simulink model "crazyflie"  (R2015b)
settings: Solver=FixedStepAuto  StartTime=0.0  StopTime=18  FixedStep=1/500  MinStep=1e-4  RelTol=1e-3
undefined symbols (not defined in the file): A, B, C, D
libraries: simulink x1
(part 1 of 3)
settings Model: NumberOfSteps=250  Creator=mattcollins  LastModifiedBy=mattcollins
settings SolverCC: AutoInsertRateTranBlk=on

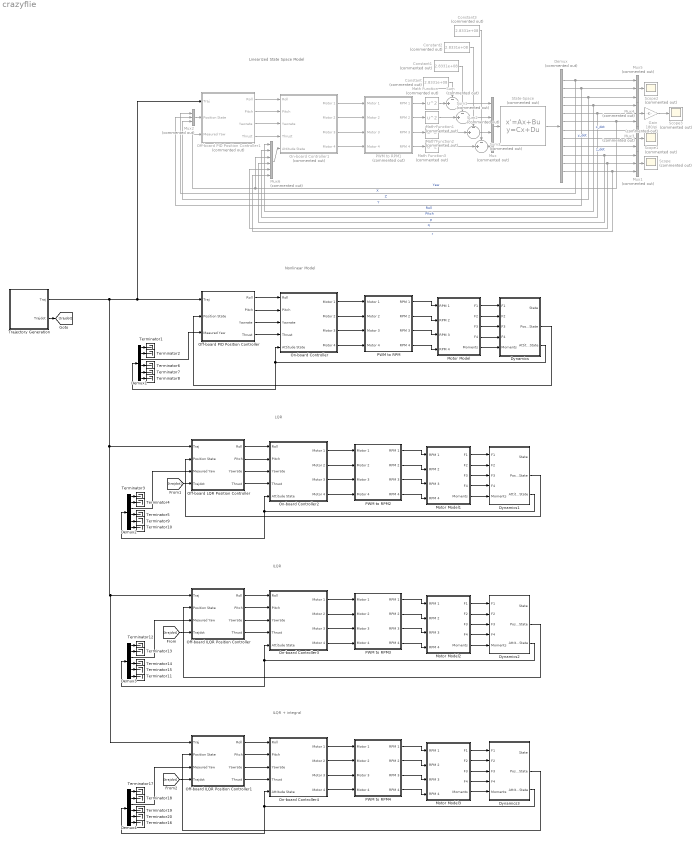
== system crazyflie ==
  note: Nonlinear Model
  note: Linearized State Space Model
  note: LQR
  note: ILQR
  note: ILQR + integral
  Constant{,1..3} (4 alike) : Constant  Commented=on  Value=2.8331e+08
  Demux : Demux  Commented=on  Outputs=12
  Demux{1..4} (4 alike) : Demux  Outputs=6
  Dynamics : Subsystem
  Dynamics1 : Subsystem
  Dynamics2 : Subsystem
  Dynamics3 : Subsystem
  Gain : Gain  Commented=on  Gain=180/pi
  Math Function{,1..3} (4 alike) : Math  Commented=on  Operator=square  SaturateOnIntegerOverflow=on
  Motor Model : Subsystem
  Motor Model1 : Subsystem
  Motor Model2 : Subsystem
  Motor Model3 : Subsystem
  Mux : Mux  Commented=on
  Mux{1..5} (5 alike) : Mux  Commented=on  Inputs=3
  Mux6 : Mux  Commented=on  Inputs=6
  Off-board ILQR Position Controller : Subsystem
  Off-board ILQR Position Controller1 : Subsystem
  "Off-board LQR Position Controller " : Subsystem
  Off-board PID Position Controller : Subsystem
  Off-board PID Position Controller1 : Subsystem  Commented=on
  On-board Controller : Subsystem
  On-board Controller1 : Subsystem  Commented=on
  On-board Controller2 : Subsystem
  On-board Controller3 : Subsystem
  On-board Controller4 : Subsystem
  PWM to RPM : Subsystem
  PWM to RPM1 : Subsystem  Commented=on
  PWM to RPM2 : Subsystem
  PWM to RPM3 : Subsystem
  PWM to RPM4 : Subsystem
  Scope{,1..3} (4 alike) : Scope  Commented=on
  State-Space : StateSpace  Commented=on  A=A  B=B  C=C  D=D  X0=[0;0;1;0;0;0;0;0;0;0;0;0]
  Sum{,1..3} (4 alike) : Sum  Commented=on  Inputs=-|+||
  Terminator{1..20} (20 alike) : Terminator
  Trajectory Generation : Subsystem
  wires:
  On-board Controller/1(Motor 1) -> PWM to RPM/1(Motor 1)
  On-board Controller/2(Motor 2) -> PWM to RPM/2(Motor 2)
  On-board Controller/3(Motor 3) -> PWM to RPM/3(Motor 3)
  On-board Controller/4(Motor 4) -> PWM to RPM/4(Motor 4)
  PWM to RPM/1(RPM 1) -> Motor Model/1(RPM 1)
  PWM to RPM/2(RPM 2) -> Motor Model/2(RPM 2)
  PWM to RPM/3(RPM 3) -> Motor Model/3(RPM 3)
  PWM to RPM/4(RPM 4) -> Motor Model/4(RPM 4)
  Motor Model/1(F1) -> Dynamics/1(F1)
  Dynamics/3(Attitude State) -> On-board Controller/5(Attitude State), Demux1/1
  Off-board PID Position Controller/1(Roll) -> On-board Controller/1(Roll)
  Off-board PID Position Controller/2(Pitch) -> On-board Controller/2(Pitch)
  Off-board PID Position Controller/3(Yawrate) -> On-board Controller/3(Yawrate)
  Off-board PID Position Controller/4(Thrust) -> On-board Controller/4(Thrust)
  Motor Model/2(F2) -> Dynamics/2(F2)
  Motor Model/3(F3) -> Dynamics/3(F3)
  Motor Model/4(F4) -> Dynamics/4(F4)
  Motor Model/5(Moments) -> Dynamics/5(Moments)
  Demux1/3 -> Off-board PID Position Controller/3(Meaured Yaw)
  Demux1/1 -> Terminator1/1
  Demux1/2 -> Terminator2/1
  Demux1/4 -> Terminator6/1
  Demux1/5 -> Terminator7/1
  Demux1/6 -> Terminator8/1
  State-Space/1 -> Demux/1
  Demux/10 -> Mux6/4, Mux1/1  "p"
  Demux/11 -> Mux6/5, Mux1/2  "q"
  Demux/12 -> Mux6/6, Mux1/3  "r"
  Mux1/1 -> Scope/1
  Mux3/1 -> Scope1/1
  Demux/7 -> Mux3/1  "x_dot"
  Demux/8 -> Mux3/2  "y_dot"
  Demux/9 -> Mux3/3  "z_dot"
  Demux/4 -> Mux6/1, Mux4/1  "Roll"
  Demux/5 -> Mux6/2, Mux4/2  "Pitch"
  Demux/6 -> Mux6/3, Off-board PID Position Controller1/3(Meaured Yaw), Mux4/3  "Yaw"
  Demux/1 -> Mux2/1, Mux5/1  "X"
  Demux/2 -> Mux2/2, Mux5/2  "Y"
  Demux/3 -> Mux2/3, Mux5/3  "Z"
  Mux4/1 -> Gain/1
  Mux5/1 -> Scope2/1
  PWM to RPM1/1(RPM 1) -> Math Function/1
  PWM to RPM1/2(RPM 2) -> Math Function1/1
  PWM to RPM1/3(RPM 3) -> Math Function2/1
  PWM to RPM1/4(RPM 4) -> Math Function3/1
  On-board Controller1/2(Motor 2) -> PWM to RPM1/2(Motor 2)
  On-board Controller1/3(Motor 3) -> PWM to RPM1/3(Motor 3)
  On-board Controller1/4(Motor 4) -> PWM to RPM1/4(Motor 4)
  Off-board PID Position Controller1/1(Roll) -> On-board Controller1/1(Roll)
  Off-board PID Position Controller1/2(Pitch) -> On-board Controller1/2(Pitch)
  Off-board PID Position Controller1/3(Yawrate) -> On-board Controller1/3(Yawrate)
  Off-board PID Position Controller1/4(Thrust) -> On-board Controller1/4(Thrust)
  Mux2/1 -> Off-board PID Position Controller1/2(Position State)
  Mux6/1 -> On-board Controller1/5(Attitude State)
  Gain/1 -> Scope3/1
  Sum/1 -> Mux/1
  Math Function/1 -> Sum/2
  Constant/1 -> Sum/1
  Math Function3/1 -> Sum3/2
  Math Function2/1 -> Sum2/2
  Sum1/1 -> Mux/2
  Math Function1/1 -> Sum1/2
  Sum2/1 -> Mux/3
  Constant1/1 -> Sum1/1
  Constant2/1 -> Sum2/1
  Constant3/1 -> Sum3/1
  Sum3/1 -> Mux/4
  Mux/1 -> State-Space/1
  On-board Controller1/1(Motor 1) -> PWM to RPM1/1(Motor 1)
  On-board Controller2/1(Motor 1) -> PWM to RPM2/1(Motor 1)
  On-board Controller2/2(Motor 2) -> PWM to RPM2/2(Motor 2)
  On-board Controller2/3(Motor 3) -> PWM to RPM2/3(Motor 3)
  On-board Controller2/4(Motor 4) -> PWM to RPM2/4(Motor 4)
  PWM to RPM2/1(RPM 1) -> Motor Model1/1(RPM 1)
  PWM to RPM2/2(RPM 2) -> Motor Model1/2(RPM 2)
  PWM to RPM2/3(RPM 3) -> Motor Model1/3(RPM 3)
  PWM to RPM2/4(RPM 4) -> Motor Model1/4(RPM 4)
  Motor Model1/1(F1) -> Dynamics1/1(F1)
  Dynamics1/3(Attitude State) -> Demux2/1, On-board Controller2/5(Attitude State)
  "Off-board LQR Position Controller "/1(Roll) -> On-board Controller2/1(Roll)
  "Off-board LQR Position Controller "/2(Pitch) -> On-board Controller2/2(Pitch)
  "Off-board LQR Position Controller "/3(Yawrate) -> On-board Controller2/3(Yawrate)
  "Off-board LQR Position Controller "/4(Thrust) -> On-board Controller2/4(Thrust)
  Motor Model1/2(F2) -> Dynamics1/2(F2)
  Motor Model1/3(F3) -> Dynamics1/3(F3)
  Motor Model1/4(F4) -> Dynamics1/4(F4)
  Motor Model1/5(Moments) -> Dynamics1/5(Moments)
  Demux2/3 -> "Off-board LQR Position Controller "/3(Meaured Yaw)
  Demux2/1 -> Terminator3/1
  Demux2/2 -> Terminator4/1
  Demux2/4 -> Terminator5/1
  Demux2/5 -> Terminator9/1
  Demux2/6 -> Terminator10/1
  On-board Controller3/1(Motor 1) -> PWM to RPM3/1(Motor 1)
  On-board Controller3/2(Motor 2) -> PWM to RPM3/2(Motor 2)
  On-board Controller3/3(Motor 3) -> PWM to RPM3/3(Motor 3)
  On-board Controller3/4(Motor 4) -> PWM to RPM3/4(Motor 4)
  PWM to RPM3/1(RPM 1) -> Motor Model2/1(RPM 1)
  PWM to RPM3/2(RPM 2) -> Motor Model2/2(RPM 2)
  PWM to RPM3/3(RPM 3) -> Motor Model2/3(RPM 3)
  PWM to RPM3/4(RPM 4) -> Motor Model2/4(RPM 4)
  Motor Model2/1(F1) -> Dynamics2/1(F1)
  Dynamics2/3(Attitude State) -> Demux3/1, On-board Controller3/5(Attitude State)
  Off-board ILQR Position Controller/1(Roll) -> On-board Controller3/1(Roll)
  Off-board ILQR Position Controller/2(Pitch) -> On-board Controller3/2(Pitch)
  Off-board ILQR Position Controller/3(Yawrate) -> On-board Controller3/3(Yawrate)
  Off-board ILQR Position Controller/4(Thrust) -> On-board Controller3/4(Thrust)
  Motor Model2/2(F2) -> Dynamics2/2(F2)
  Motor Model2/3(F3) -> Dynamics2/3(F3)
  Motor Model2/4(F4) -> Dynamics2/4(F4)
  Motor Model2/5(Moments) -> Dynamics2/5(Moments)
  Demux3/3 -> Off-board ILQR Position Controller/3(Meaured Yaw)
  Trajectory Generation/1(Traj) -> Off-board ILQR Position Controller1/1(Traj), Off-board ILQR Position Controller/1(Traj), "Off-board LQR Position Controller "/1(Traj), Off-board PID Position Controller1/1(Traj), Off-board PID Position Controller/1(Traj)
  Demux3/1 -> Terminator12/1
  Demux3/2 -> Terminator13/1
  Demux3/4 -> Terminator14/1
  Demux3/5 -> Terminator15/1
  Demux3/6 -> Terminator11/1
  Trajectory Generation/2(Trajdot) -> [trajdot]
  [trajdot] -> Off-board ILQR Position Controller/4("Trajdot ")
  [trajdot] -> "Off-board LQR Position Controller "/4("Trajdot ")
  On-board Controller4/1(Motor 1) -> PWM to RPM4/1(Motor 1)
  On-board Controller4/2(Motor 2) -> PWM to RPM4/2(Motor 2)
  On-board Controller4/3(Motor 3) -> PWM to RPM4/3(Motor 3)
  On-board Controller4/4(Motor 4) -> PWM to RPM4/4(Motor 4)
  PWM to RPM4/1(RPM 1) -> Motor Model3/1(RPM 1)
  PWM to RPM4/2(RPM 2) -> Motor Model3/2(RPM 2)
  PWM to RPM4/3(RPM 3) -> Motor Model3/3(RPM 3)
  PWM to RPM4/4(RPM 4) -> Motor Model3/4(RPM 4)
  Motor Model3/1(F1) -> Dynamics3/1(F1)
  Dynamics3/3(Attitude State) -> Demux4/1, On-board Controller4/5(Attitude State)
  Off-board ILQR Position Controller1/1(Roll) -> On-board Controller4/1(Roll)
  Off-board ILQR Position Controller1/2(Pitch) -> On-board Controller4/2(Pitch)
  Off-board ILQR Position Controller1/3(Yawrate) -> On-board Controller4/3(Yawrate)
  Off-board ILQR Position Controller1/4(Thrust) -> On-board Controller4/4(Thrust)
  Motor Model3/2(F2) -> Dynamics3/2(F2)
  Motor Model3/3(F3) -> Dynamics3/3(F3)
  Motor Model3/4(F4) -> Dynamics3/4(F4)
  Motor Model3/5(Moments) -> Dynamics3/5(Moments)
  Demux4/3 -> Off-board ILQR Position Controller1/3(Meaured Yaw)
  Demux4/1 -> Terminator17/1
  Demux4/2 -> Terminator18/1
  Demux4/4 -> Terminator19/1
  Demux4/5 -> Terminator20/1
  Demux4/6 -> Terminator16/1
  [trajdot] -> Off-board ILQR Position Controller1/4("Trajdot ")
  Dynamics1/2(Position State) -> "Off-board LQR Position Controller "/2(Position State)
  Dynamics/2(Position State) -> Off-board PID Position Controller/2(Position State)
  Dynamics2/2(Position State) -> Off-board ILQR Position Controller/2(Position State)
  Dynamics3/2(Position State) -> Off-board ILQR Position Controller1/2(Position State)

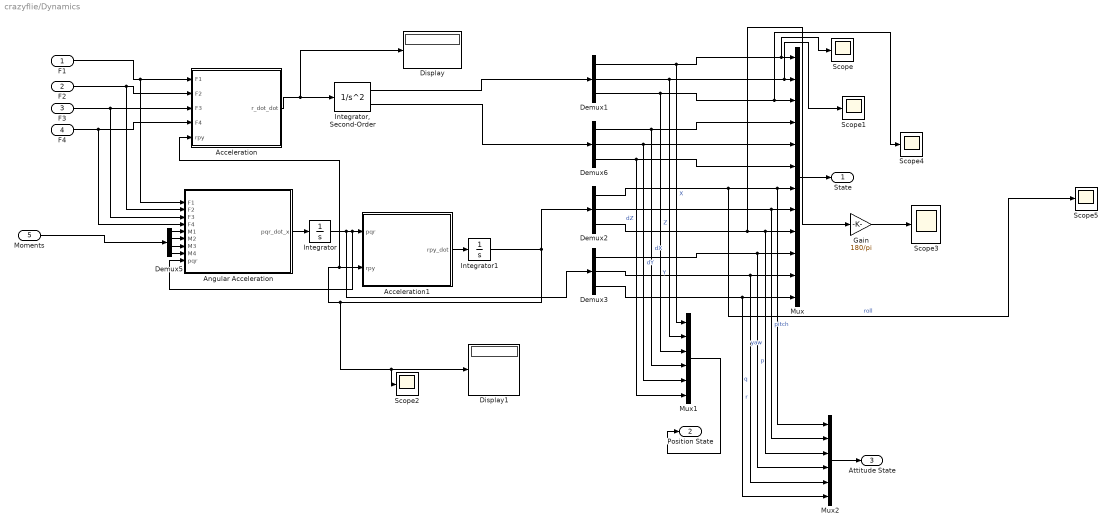
== system crazyflie/Dynamics ==
  F1 : Inport
  F2 : Inport  Port=2
  F3 : Inport  Port=3
  F4 : Inport  Port=4
  Moments : Inport  Port=5
  Acceleration : MATLAB Function  TreatAsAtomicUnit=on
  Acceleration1 : MATLAB Function  TreatAsAtomicUnit=on
  Angular Acceleration : MATLAB Function  TreatAsAtomicUnit=on
  Demux{1..3,6} (4 alike) : Demux  Outputs=3
  Demux5 : Demux
  Display : Display
  Display1 : Display
  Gain : Gain  Gain=180/pi
  Integrator : Integrator  InitialCondition=[0;0;0]
  "Integrator, Second-Order" : SecondOrderIntegrator  ICX=[0;0;0]  LimitX=on  UpperLimitX=[inf,inf,inf]  LowerLimitX=[-inf,-inf,0]  StateNameX=['x', 'y', 'z']  ICDXDT=[0;0;0]  LimitDXDT=on  UpperLimitDXDT=Inf  LowerLimitDXDT=-Inf  StateNameDXDT=['dx', 'dy', 'dz']
  Integrator1 : Integrator  InitialCondition=[0;0;0]
  Mux : Mux  Inputs=12
  Mux1 : Mux  Inputs=6
  Mux2 : Mux  Inputs=6
  Scope{,1..5} (6 alike) : Scope
  State : Outport
  Position State : Outport  Port=2
  Attitude State : Outport  Port=3
  wires:
  Demux2/1 -> Scope5/1, Mux2/1, Mux/7  "roll"
  Demux2/2 -> Mux2/2, Mux/8  "pitch"
  Demux2/3 -> Gain/1, Mux2/3, Mux/9  "yaw"
  Demux3/1 -> Mux2/4, Mux/10  "p"
  Demux3/2 -> Mux2/5, Mux/11  "q"
  Demux3/3 -> Mux2/6, Mux/12  "r"
  Mux/1 -> State/1
  Mux1/1 -> Position State/1
  Mux2/1 -> Attitude State/1
  Demux5/1 -> Angular Acceleration/5(M1)
  Demux5/2 -> Angular Acceleration/6(M2)
  Demux5/3 -> Angular Acceleration/7(M3)
  Demux5/4 -> Angular Acceleration/8(M4)
  Angular Acceleration/1(pqr_dot_x) -> Integrator/1
  Integrator/1 -> Demux3/1, Angular Acceleration/9(pqr), Acceleration1/1(pqr)
  Acceleration1/1(rpy_dot) -> Integrator1/1
  Integrator1/1 -> Demux2/1, Scope2/1, Display1/1, Acceleration/5(rpy), Acceleration1/2(rpy)
  Acceleration/1(r_dot_dot) -> Display/1, "Integrator, Second-Order"/1
  "Integrator, Second-Order"/1 -> Demux1/1
  "Integrator, Second-Order"/2 -> Demux6/1
  Demux1/1 -> Mux1/1, Scope/1, Mux/1  "X"
  Demux1/2 -> Mux1/2, Scope1/1, Mux/2  "Y"
  Demux1/3 -> Mux1/3, Scope4/1, Mux/3  "Z"
  Demux6/1 -> Mux1/4, Mux/4  "dX"
  Demux6/2 -> Mux1/5, Mux/5  "dY"
  Demux6/3 -> Mux1/6, Mux/6  "dZ"
  Moments/1 -> Demux5/1
  F2/1 -> Angular Acceleration/2(F2), Acceleration/2(F2)
  F3/1 -> Angular Acceleration/3(F3), Acceleration/3(F3)
  F4/1 -> Angular Acceleration/4(F4), Acceleration/4(F4)
  F1/1 -> Angular Acceleration/1(F1), Acceleration/1(F1)
  Gain/1 -> Scope3/1

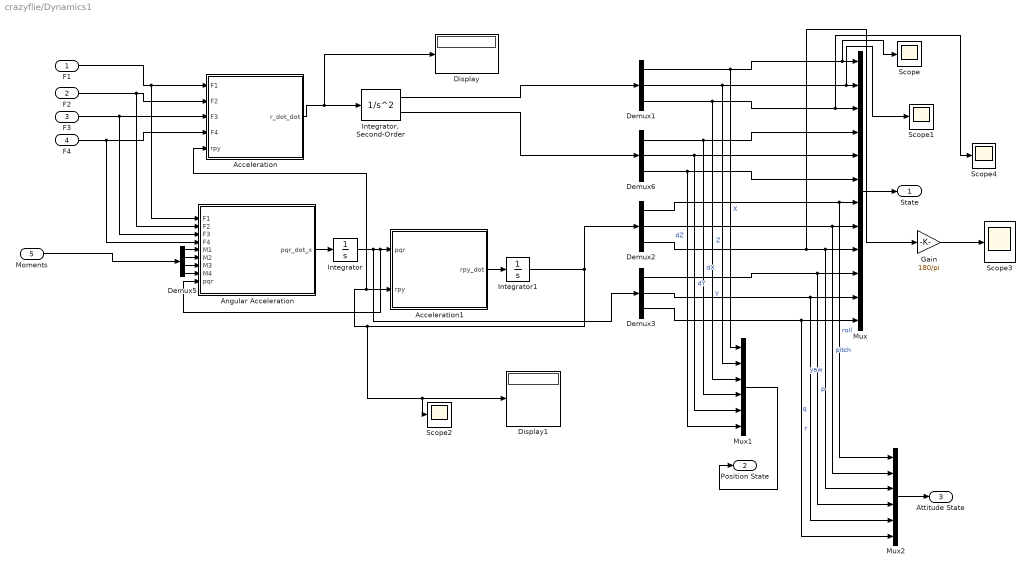
== system crazyflie/Dynamics1 ==
  F1 : Inport
  F2 : Inport  Port=2
  F3 : Inport  Port=3
  F4 : Inport  Port=4
  Moments : Inport  Port=5
  Acceleration : MATLAB Function  TreatAsAtomicUnit=on
  Acceleration1 : MATLAB Function  TreatAsAtomicUnit=on
  Angular Acceleration : MATLAB Function  TreatAsAtomicUnit=on
  Demux{1..3,6} (4 alike) : Demux  Outputs=3
  Demux5 : Demux
  Display : Display
  Display1 : Display
  Gain : Gain  Gain=180/pi
  Integrator : Integrator  InitialCondition=[0;0;0]
  "Integrator, Second-Order" : SecondOrderIntegrator  ICX=[0;0;0]  LimitX=on  UpperLimitX=[inf,inf,inf]  LowerLimitX=[-inf,-inf,0]  StateNameX=['x', 'y', 'z']  ICDXDT=[0;0;0]  LimitDXDT=on  UpperLimitDXDT=Inf  LowerLimitDXDT=-Inf  StateNameDXDT=['dx', 'dy', 'dz']
  Integrator1 : Integrator  InitialCondition=[0;0;0]
  Mux : Mux  Inputs=12
  Mux1 : Mux  Inputs=6
  Mux2 : Mux  Inputs=6
  Scope{,1..4} (5 alike) : Scope
  State : Outport
  Position State : Outport  Port=2
  Attitude State : Outport  Port=3
  wires:
  Demux2/1 -> Mux2/1, Mux/7  "roll"
  Demux2/2 -> Mux2/2, Mux/8  "pitch"
  Demux2/3 -> Gain/1, Mux2/3, Mux/9  "yaw"
  Demux3/1 -> Mux2/4, Mux/10  "p"
  Demux3/2 -> Mux2/5, Mux/11  "q"
  Demux3/3 -> Mux2/6, Mux/12  "r"
  Mux/1 -> State/1
  Mux1/1 -> Position State/1
  Mux2/1 -> Attitude State/1
  Demux5/1 -> Angular Acceleration/5(M1)
  Demux5/2 -> Angular Acceleration/6(M2)
  Demux5/3 -> Angular Acceleration/7(M3)
  Demux5/4 -> Angular Acceleration/8(M4)
  Angular Acceleration/1(pqr_dot_x) -> Integrator/1
  Integrator/1 -> Demux3/1, Angular Acceleration/9(pqr), Acceleration1/1(pqr)
  Acceleration1/1(rpy_dot) -> Integrator1/1
  Integrator1/1 -> Demux2/1, Scope2/1, Display1/1, Acceleration/5(rpy), Acceleration1/2(rpy)
  Acceleration/1(r_dot_dot) -> Display/1, "Integrator, Second-Order"/1
  "Integrator, Second-Order"/1 -> Demux1/1
  "Integrator, Second-Order"/2 -> Demux6/1
  Demux1/1 -> Mux1/1, Scope/1, Mux/1  "X"
  Demux1/2 -> Mux1/2, Scope1/1, Mux/2  "Y"
  Demux1/3 -> Mux1/3, Scope4/1, Mux/3  "Z"
  Demux6/1 -> Mux1/4, Mux/4  "dX"
  Demux6/2 -> Mux1/5, Mux/5  "dY"
  Demux6/3 -> Mux1/6, Mux/6  "dZ"
  Moments/1 -> Demux5/1
  F2/1 -> Angular Acceleration/2(F2), Acceleration/2(F2)
  F3/1 -> Angular Acceleration/3(F3), Acceleration/3(F3)
  F4/1 -> Angular Acceleration/4(F4), Acceleration/4(F4)
  F1/1 -> Angular Acceleration/1(F1), Acceleration/1(F1)
  Gain/1 -> Scope3/1

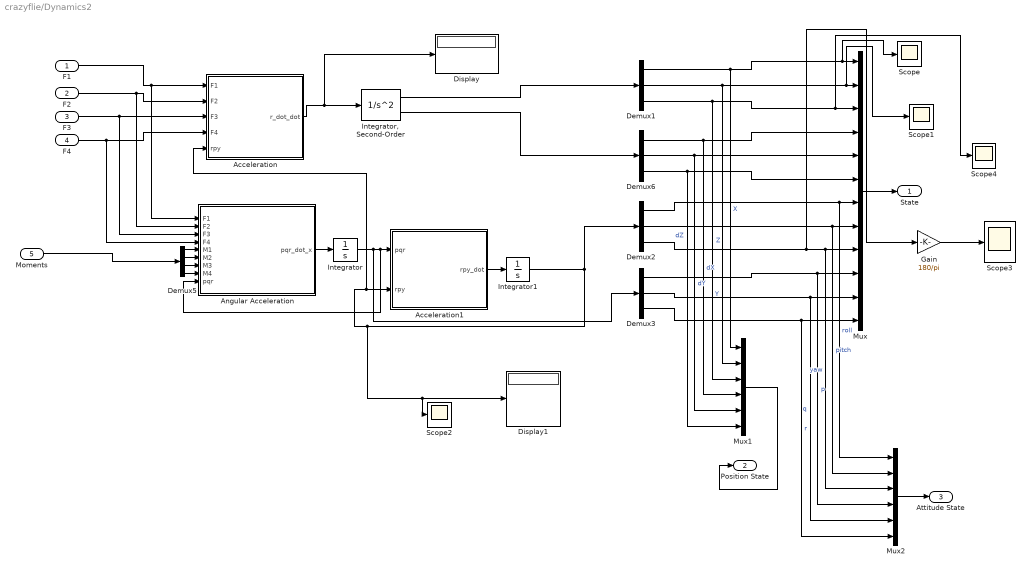
== system crazyflie/Dynamics2 ==
  F1 : Inport
  F2 : Inport  Port=2
  F3 : Inport  Port=3
  F4 : Inport  Port=4
  Moments : Inport  Port=5
  Acceleration : MATLAB Function  TreatAsAtomicUnit=on
  Acceleration1 : MATLAB Function  TreatAsAtomicUnit=on
  Angular Acceleration : MATLAB Function  TreatAsAtomicUnit=on
  Demux{1..3,6} (4 alike) : Demux  Outputs=3
  Demux5 : Demux
  Display : Display
  Display1 : Display
  Gain : Gain  Gain=180/pi
  Integrator : Integrator  InitialCondition=[0;0;0]
  "Integrator, Second-Order" : SecondOrderIntegrator  ICX=[0;0;0]  LimitX=on  UpperLimitX=[inf,inf,inf]  LowerLimitX=[-inf,-inf,0]  StateNameX=['x', 'y', 'z']  ICDXDT=[0;0;0]  LimitDXDT=on  UpperLimitDXDT=Inf  LowerLimitDXDT=-Inf  StateNameDXDT=['dx', 'dy', 'dz']
  Integrator1 : Integrator  InitialCondition=[0;0;0]
  Mux : Mux  Inputs=12
  Mux1 : Mux  Inputs=6
  Mux2 : Mux  Inputs=6
  Scope{,1..4} (5 alike) : Scope
  State : Outport
  Position State : Outport  Port=2
  Attitude State : Outport  Port=3
  wires:
  Demux2/1 -> Mux2/1, Mux/7  "roll"
  Demux2/2 -> Mux2/2, Mux/8  "pitch"
  Demux2/3 -> Gain/1, Mux2/3, Mux/9  "yaw"
  Demux3/1 -> Mux2/4, Mux/10  "p"
  Demux3/2 -> Mux2/5, Mux/11  "q"
  Demux3/3 -> Mux2/6, Mux/12  "r"
  Mux/1 -> State/1
  Mux1/1 -> Position State/1
  Mux2/1 -> Attitude State/1
  Demux5/1 -> Angular Acceleration/5(M1)
  Demux5/2 -> Angular Acceleration/6(M2)
  Demux5/3 -> Angular Acceleration/7(M3)
  Demux5/4 -> Angular Acceleration/8(M4)
  Angular Acceleration/1(pqr_dot_x) -> Integrator/1
  Integrator/1 -> Demux3/1, Angular Acceleration/9(pqr), Acceleration1/1(pqr)
  Acceleration1/1(rpy_dot) -> Integrator1/1
  Integrator1/1 -> Demux2/1, Scope2/1, Display1/1, Acceleration/5(rpy), Acceleration1/2(rpy)
  Acceleration/1(r_dot_dot) -> Display/1, "Integrator, Second-Order"/1
  "Integrator, Second-Order"/1 -> Demux1/1
  "Integrator, Second-Order"/2 -> Demux6/1
  Demux1/1 -> Mux1/1, Scope/1, Mux/1  "X"
  Demux1/2 -> Mux1/2, Scope1/1, Mux/2  "Y"
  Demux1/3 -> Mux1/3, Scope4/1, Mux/3  "Z"
  Demux6/1 -> Mux1/4, Mux/4  "dX"
  Demux6/2 -> Mux1/5, Mux/5  "dY"
  Demux6/3 -> Mux1/6, Mux/6  "dZ"
  Moments/1 -> Demux5/1
  F2/1 -> Angular Acceleration/2(F2), Acceleration/2(F2)
  F3/1 -> Angular Acceleration/3(F3), Acceleration/3(F3)
  F4/1 -> Angular Acceleration/4(F4), Acceleration/4(F4)
  F1/1 -> Angular Acceleration/1(F1), Acceleration/1(F1)
  Gain/1 -> Scope3/1

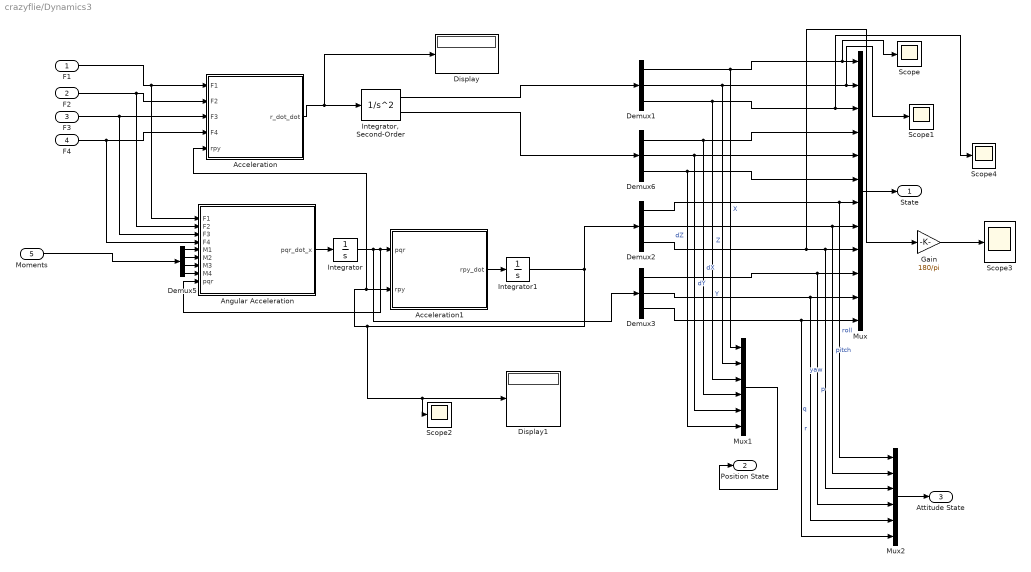
== system crazyflie/Dynamics3 ==
  F1 : Inport
  F2 : Inport  Port=2
  F3 : Inport  Port=3
  F4 : Inport  Port=4
  Moments : Inport  Port=5
  Acceleration : MATLAB Function  TreatAsAtomicUnit=on
  Acceleration1 : MATLAB Function  TreatAsAtomicUnit=on
  Angular Acceleration : MATLAB Function  TreatAsAtomicUnit=on
  Demux{1..3,6} (4 alike) : Demux  Outputs=3
  Demux5 : Demux
  Display : Display
  Display1 : Display
  Gain : Gain  Gain=180/pi
  Integrator : Integrator  InitialCondition=[0;0;0]
  "Integrator, Second-Order" : SecondOrderIntegrator  ICX=[0;0;0]  LimitX=on  UpperLimitX=[inf,inf,inf]  LowerLimitX=[-inf,-inf,0]  StateNameX=['x', 'y', 'z']  ICDXDT=[0;0;0]  LimitDXDT=on  UpperLimitDXDT=Inf  LowerLimitDXDT=-Inf  StateNameDXDT=['dx', 'dy', 'dz']
  Integrator1 : Integrator  InitialCondition=[0;0;0]
  Mux : Mux  Inputs=12
  Mux1 : Mux  Inputs=6
  Mux2 : Mux  Inputs=6
  Scope{,1..4} (5 alike) : Scope
  State : Outport
  Position State : Outport  Port=2
  Attitude State : Outport  Port=3
  wires:
  Demux2/1 -> Mux2/1, Mux/7  "roll"
  Demux2/2 -> Mux2/2, Mux/8  "pitch"
  Demux2/3 -> Gain/1, Mux2/3, Mux/9  "yaw"
  Demux3/1 -> Mux2/4, Mux/10  "p"
  Demux3/2 -> Mux2/5, Mux/11  "q"
  Demux3/3 -> Mux2/6, Mux/12  "r"
  Mux/1 -> State/1
  Mux1/1 -> Position State/1
  Mux2/1 -> Attitude State/1
  Demux5/1 -> Angular Acceleration/5(M1)
  Demux5/2 -> Angular Acceleration/6(M2)
  Demux5/3 -> Angular Acceleration/7(M3)
  Demux5/4 -> Angular Acceleration/8(M4)
  Angular Acceleration/1(pqr_dot_x) -> Integrator/1
  Integrator/1 -> Demux3/1, Angular Acceleration/9(pqr), Acceleration1/1(pqr)
  Acceleration1/1(rpy_dot) -> Integrator1/1
  Integrator1/1 -> Demux2/1, Scope2/1, Display1/1, Acceleration/5(rpy), Acceleration1/2(rpy)
  Acceleration/1(r_dot_dot) -> Display/1, "Integrator, Second-Order"/1
  "Integrator, Second-Order"/1 -> Demux1/1
  "Integrator, Second-Order"/2 -> Demux6/1
  Demux1/1 -> Mux1/1, Scope/1, Mux/1  "X"
  Demux1/2 -> Mux1/2, Scope1/1, Mux/2  "Y"
  Demux1/3 -> Mux1/3, Scope4/1, Mux/3  "Z"
  Demux6/1 -> Mux1/4, Mux/4  "dX"
  Demux6/2 -> Mux1/5, Mux/5  "dY"
  Demux6/3 -> Mux1/6, Mux/6  "dZ"
  Moments/1 -> Demux5/1
  F2/1 -> Angular Acceleration/2(F2), Acceleration/2(F2)
  F3/1 -> Angular Acceleration/3(F3), Acceleration/3(F3)
  F4/1 -> Angular Acceleration/4(F4), Acceleration/4(F4)
  F1/1 -> Angular Acceleration/1(F1), Acceleration/1(F1)
  Gain/1 -> Scope3/1

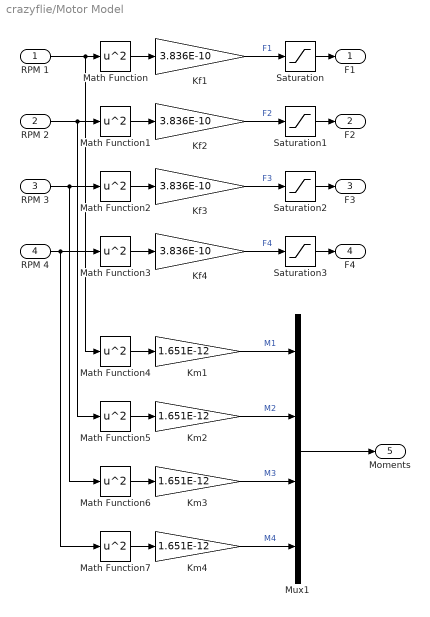
== system crazyflie/Motor Model ==
  RPM 1 : Inport
  RPM 2 : Inport  Port=2
  RPM 3 : Inport  Port=3
  RPM 4 : Inport  Port=4
  Kf{1..4} (4 alike) : Gain  Gain=3.836E-10
  Km{1..4} (4 alike) : Gain  Gain=1.651E-12
  Math Function{,1..7} (8 alike) : Math  Operator=square  SaturateOnIntegerOverflow=on
  Mux1 : Mux
  Saturation{,1..3} (4 alike) : Saturate  UpperLimit=.2  LowerLimit=0
  F1 : Outport
  F2 : Outport  Port=2
  F3 : Outport  Port=3
  F4 : Outport  Port=4
  Moments : Outport  Port=5
  wires:
  RPM 4/1 -> Math Function7/1, Math Function3/1
  RPM 3/1 -> Math Function6/1, Math Function2/1
  RPM 2/1 -> Math Function5/1, Math Function1/1
  RPM 1/1 -> Math Function4/1, Math Function/1
  Math Function/1 -> Kf1/1
  Math Function1/1 -> Kf2/1
  Math Function2/1 -> Kf3/1
  Math Function3/1 -> Kf4/1
  Kf3/1 -> Saturation2/1  "F3"
  Math Function4/1 -> Km1/1
  Math Function5/1 -> Km2/1
  Math Function6/1 -> Km3/1
  Math Function7/1 -> Km4/1
  Km4/1 -> Mux1/4  "M4"
  Km3/1 -> Mux1/3  "M3"
  Km2/1 -> Mux1/2  "M2"
  Km1/1 -> Mux1/1  "M1"
  Mux1/1 -> Moments/1
  Kf2/1 -> Saturation1/1  "F2"
  Kf1/1 -> Saturation/1  "F1"
  Kf4/1 -> Saturation3/1  "F4"
  Saturation/1 -> F1/1
  Saturation1/1 -> F2/1
  Saturation2/1 -> F3/1
  Saturation3/1 -> F4/1

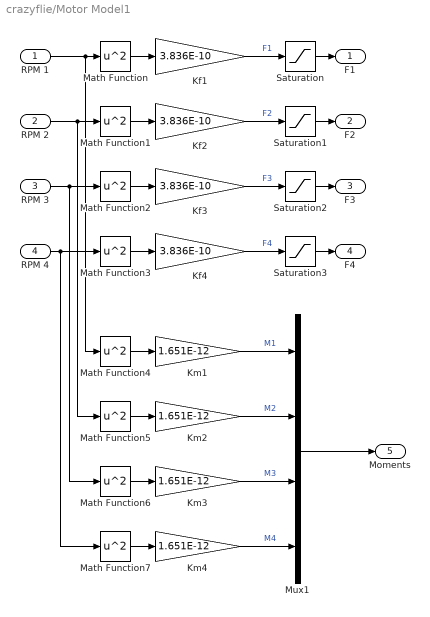
== system crazyflie/Motor Model1 ==
  RPM 1 : Inport
  RPM 2 : Inport  Port=2
  RPM 3 : Inport  Port=3
  RPM 4 : Inport  Port=4
  Kf{1..4} (4 alike) : Gain  Gain=3.836E-10
  Km{1..4} (4 alike) : Gain  Gain=1.651E-12
  Math Function{,1..7} (8 alike) : Math  Operator=square  SaturateOnIntegerOverflow=on
  Mux1 : Mux
  Saturation{,1..3} (4 alike) : Saturate  UpperLimit=.2  LowerLimit=0
  F1 : Outport
  F2 : Outport  Port=2
  F3 : Outport  Port=3
  F4 : Outport  Port=4
  Moments : Outport  Port=5
  wires:
  RPM 4/1 -> Math Function7/1, Math Function3/1
  RPM 3/1 -> Math Function6/1, Math Function2/1
  RPM 2/1 -> Math Function5/1, Math Function1/1
  RPM 1/1 -> Math Function4/1, Math Function/1
  Math Function/1 -> Kf1/1
  Math Function1/1 -> Kf2/1
  Math Function2/1 -> Kf3/1
  Math Function3/1 -> Kf4/1
  Kf3/1 -> Saturation2/1  "F3"
  Math Function4/1 -> Km1/1
  Math Function5/1 -> Km2/1
  Math Function6/1 -> Km3/1
  Math Function7/1 -> Km4/1
  Km4/1 -> Mux1/4  "M4"
  Km3/1 -> Mux1/3  "M3"
  Km2/1 -> Mux1/2  "M2"
  Km1/1 -> Mux1/1  "M1"
  Mux1/1 -> Moments/1
  Kf2/1 -> Saturation1/1  "F2"
  Kf1/1 -> Saturation/1  "F1"
  Kf4/1 -> Saturation3/1  "F4"
  Saturation/1 -> F1/1
  Saturation1/1 -> F2/1
  Saturation2/1 -> F3/1
  Saturation3/1 -> F4/1

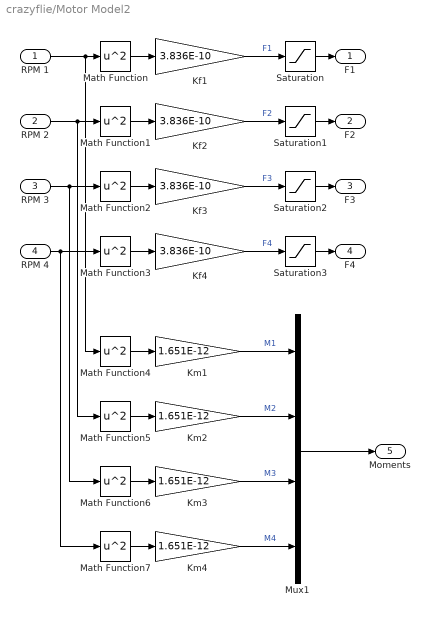
== system crazyflie/Motor Model2 ==
  RPM 1 : Inport
  RPM 2 : Inport  Port=2
  RPM 3 : Inport  Port=3
  RPM 4 : Inport  Port=4
  Kf{1..4} (4 alike) : Gain  Gain=3.836E-10
  Km{1..4} (4 alike) : Gain  Gain=1.651E-12
  Math Function{,1..7} (8 alike) : Math  Operator=square  SaturateOnIntegerOverflow=on
  Mux1 : Mux
  Saturation{,1..3} (4 alike) : Saturate  UpperLimit=.2  LowerLimit=0
  F1 : Outport
  F2 : Outport  Port=2
  F3 : Outport  Port=3
  F4 : Outport  Port=4
  Moments : Outport  Port=5
  wires:
  RPM 4/1 -> Math Function7/1, Math Function3/1
  RPM 3/1 -> Math Function6/1, Math Function2/1
  RPM 2/1 -> Math Function5/1, Math Function1/1
  RPM 1/1 -> Math Function4/1, Math Function/1
  Math Function/1 -> Kf1/1
  Math Function1/1 -> Kf2/1
  Math Function2/1 -> Kf3/1
  Math Function3/1 -> Kf4/1
  Kf3/1 -> Saturation2/1  "F3"
  Math Function4/1 -> Km1/1
  Math Function5/1 -> Km2/1
  Math Function6/1 -> Km3/1
  Math Function7/1 -> Km4/1
  Km4/1 -> Mux1/4  "M4"
  Km3/1 -> Mux1/3  "M3"
  Km2/1 -> Mux1/2  "M2"
  Km1/1 -> Mux1/1  "M1"
  Mux1/1 -> Moments/1
  Kf2/1 -> Saturation1/1  "F2"
  Kf1/1 -> Saturation/1  "F1"
  Kf4/1 -> Saturation3/1  "F4"
  Saturation/1 -> F1/1
  Saturation1/1 -> F2/1
  Saturation2/1 -> F3/1
  Saturation3/1 -> F4/1

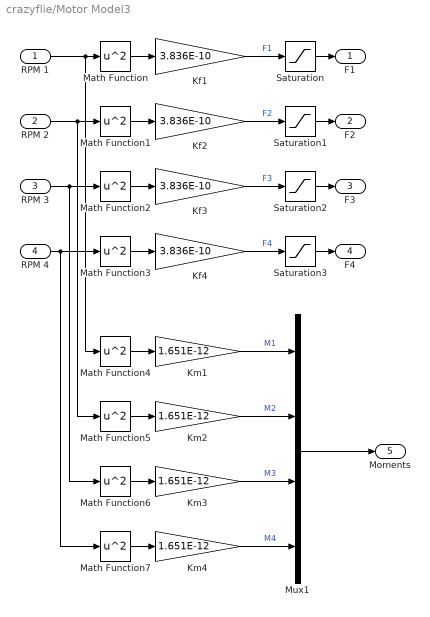
== system crazyflie/Motor Model3 ==
  RPM 1 : Inport
  RPM 2 : Inport  Port=2
  RPM 3 : Inport  Port=3
  RPM 4 : Inport  Port=4
  Kf{1..4} (4 alike) : Gain  Gain=3.836E-10
  Km{1..4} (4 alike) : Gain  Gain=1.651E-12
  Math Function{,1..7} (8 alike) : Math  Operator=square  SaturateOnIntegerOverflow=on
  Mux1 : Mux
  Saturation{,1..3} (4 alike) : Saturate  UpperLimit=.2  LowerLimit=0
  F1 : Outport
  F2 : Outport  Port=2
  F3 : Outport  Port=3
  F4 : Outport  Port=4
  Moments : Outport  Port=5
  wires:
  RPM 4/1 -> Math Function7/1, Math Function3/1
  RPM 3/1 -> Math Function6/1, Math Function2/1
  RPM 2/1 -> Math Function5/1, Math Function1/1
  RPM 1/1 -> Math Function4/1, Math Function/1
  Math Function/1 -> Kf1/1
  Math Function1/1 -> Kf2/1
  Math Function2/1 -> Kf3/1
  Math Function3/1 -> Kf4/1
  Kf3/1 -> Saturation2/1  "F3"
  Math Function4/1 -> Km1/1
  Math Function5/1 -> Km2/1
  Math Function6/1 -> Km3/1
  Math Function7/1 -> Km4/1
  Km4/1 -> Mux1/4  "M4"
  Km3/1 -> Mux1/3  "M3"
  Km2/1 -> Mux1/2  "M2"
  Km1/1 -> Mux1/1  "M1"
  Mux1/1 -> Moments/1
  Kf2/1 -> Saturation1/1  "F2"
  Kf1/1 -> Saturation/1  "F1"
  Kf4/1 -> Saturation3/1  "F4"
  Saturation/1 -> F1/1
  Saturation1/1 -> F2/1
  Saturation2/1 -> F3/1
  Saturation3/1 -> F4/1

== system crazyflie/Off-board ILQR Position Controller ==
  Traj : Inport
  Position State : Inport  Port=2
  Meaured Yaw : Inport  Port=3
  "Trajdot " : Inport  Port=4
  Demux1 : Demux  Outputs=6
  Display : Display
  Gain1 : Gain
  Gain2 : Gain  Gain=180/pi
  ILQR : Subsystem
  Saturation : Saturate  UpperLimit=60000  LowerLimit=1000
  Saturation1 : Saturate  UpperLimit=30  LowerLimit=-30
  Saturation2 : Saturate  UpperLimit=30  LowerLimit=-30
  Scope : Scope
  Scope1 : Scope
  Subsystem2 : Subsystem
  Roll : Outport
  Pitch : Outport  Port=2
  Yawrate : Outport  Port=3
  Thrust : Outport  Port=4
  wires:
  Position State/1 -> Demux1/1
  ILQR/4(Thrust Desired) -> Saturation/1
  Saturation/1 -> Display/1, Thrust/1
  Saturation2/1 -> Scope/1, Roll/1
  ILQR/3(Yaw rate Desired) -> Gain1/1
  ILQR/1(Roll Desired) -> Subsystem2/1(Rollw)
  ILQR/2(Pitch Desired) -> Subsystem2/2(Pitchw)
  Subsystem2/1(Rollb Error) -> Saturation1/1
  Subsystem2/2(Pitchb Error) -> Saturation2/1
  Traj/1 -> ILQR/8(traj)
  "Trajdot "/1 -> ILQR/9(trajdot)
  Demux1/1 -> ILQR/1(x meas)  "Mesured X"
  Demux1/2 -> ILQR/2(y meas)  "Measured Y"
  Demux1/3 -> ILQR/3(z meas)  "Measured Z"
  Demux1/4 -> ILQR/4(xdot meas)  "Measured Xdot"
  Demux1/5 -> ILQR/5(ydot meas)  "Measured Ydot"
  Demux1/6 -> ILQR/6(zdot meas)  "Measured Zdot"
  Meaured Yaw/1 -> [yaw], Gain2/1
  [yaw] -> Subsystem2/3(Measured Yaw)
  Gain1/1 -> Yawrate/1
  Gain2/1 -> ILQR/7("yaw meas ")
  Saturation1/1 -> Scope1/1, Pitch/1

== system crazyflie/Off-board ILQR Position Controller1 ==
  Traj : Inport
  Position State : Inport  Port=2
  Meaured Yaw : Inport  Port=3
  "Trajdot " : Inport  Port=4
  Demux : Demux
  Demux1 : Demux  Outputs=6
  Display : Display
  Gain1 : Gain
  Gain2 : Gain  Gain=180/pi
  ILQR : Subsystem
  Integrator : Integrator
  Integrator1 : Integrator
  Integrator2 : Integrator
  Saturation : Saturate  UpperLimit=60000  LowerLimit=1000
  Saturation1 : Saturate  UpperLimit=30  LowerLimit=-30
  Saturation2 : Saturate  UpperLimit=30  LowerLimit=-30
  Scope : Scope
  Scope1 : Scope
  Subsystem2 : Subsystem
  Subtract : Sum  Inputs=+-
  Subtract1 : Sum  Inputs=+-
  Subtract2 : Sum  Inputs=+-
  Roll : Outport
  Pitch : Outport  Port=2
  Yawrate : Outport  Port=3
  Thrust : Outport  Port=4
  wires:
  Position State/1 -> Demux1/1
  ILQR/4(Thrust Desired) -> Saturation/1
  Saturation/1 -> Display/1, Thrust/1
  Saturation2/1 -> Scope/1, Roll/1
  ILQR/3(Yaw rate Desired) -> Gain1/1
  ILQR/1(Roll Desired) -> Subsystem2/1(Rollw)
  ILQR/2(Pitch Desired) -> Subsystem2/2(Pitchw)
  Subsystem2/1(Rollb Error) -> Saturation1/1
  Subsystem2/2(Pitchb Error) -> Saturation2/1
  Traj/1 -> Demux/1, ILQR/8(traj)
  "Trajdot "/1 -> ILQR/9(trajdot)
  Demux1/1 -> Subtract/2, ILQR/1(x meas)  "Mesured X"
  Demux1/2 -> Subtract1/2, ILQR/2(y meas)  "Measured Y"
  Demux1/3 -> Subtract2/2, ILQR/3(z meas)  "Measured Z"
  Demux1/4 -> ILQR/4(xdot meas)  "Measured Xdot"
  Demux1/5 -> ILQR/5(ydot meas)  "Measured Ydot"
  Demux1/6 -> ILQR/6(zdot meas)  "Measured Zdot"
  Meaured Yaw/1 -> [yaw], Gain2/1
  [yaw] -> Subsystem2/3(Measured Yaw)
  Gain1/1 -> Yawrate/1
  Gain2/1 -> ILQR/7("yaw meas ")
  Saturation1/1 -> Scope1/1, Pitch/1
  Demux/1 -> Subtract/1
  Demux/2 -> Subtract1/1
  Demux/3 -> Subtract2/1
  Subtract2/1 -> Integrator/1
  Integrator/1 -> ILQR/12(zerr)
  Subtract1/1 -> Integrator1/1
  Integrator1/1 -> ILQR/11(yerr)
  Subtract/1 -> Integrator2/1
  Integrator2/1 -> ILQR/10(xerr)

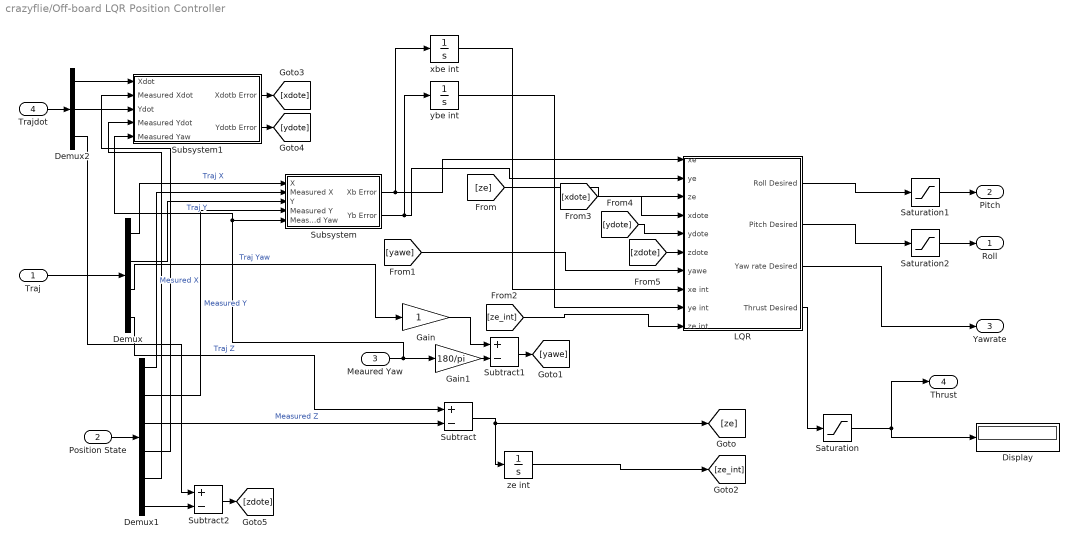
== system crazyflie/Off-board LQR Position Controller  ==
  Traj : Inport
  Position State : Inport  Port=2
  Meaured Yaw : Inport  Port=3
  "Trajdot " : Inport  Port=4
  Demux : Demux
  Demux1 : Demux  Outputs=6
  Demux2 : Demux  Outputs=3
  Display : Display
  Gain : Gain
  Gain1 : Gain  Gain=180/pi
  LQR : Subsystem
  Saturation : Saturate  UpperLimit=60000  LowerLimit=1000
  Saturation1 : Saturate  UpperLimit=30  LowerLimit=-30
  Saturation2 : Saturate  UpperLimit=30  LowerLimit=-30
  Subsystem : Subsystem
  Subsystem1 : Subsystem
  Subtract : Sum  Inputs=+-
  Subtract1 : Sum  Inputs=+-
  Subtract2 : Sum  Inputs=+-
  xbe int : Integrator
  ybe int : Integrator
  ze int : Integrator  LimitOutput=on  UpperSaturationLimit=5  LowerSaturationLimit=-5
  Roll : Outport
  Pitch : Outport  Port=2
  Yawrate : Outport  Port=3
  Thrust : Outport  Port=4
  wires:
  Traj/1 -> Demux/1
  LQR/1(Roll Desired) -> Saturation1/1
  Demux/4 -> Subtract/1  "Traj Z"
  Demux/3 -> Gain/1  "Traj Yaw"
  Position State/1 -> Demux1/1
  Demux1/3 -> Subtract/2  "Measured Z"
  LQR/2(Pitch Desired) -> Saturation2/1
  LQR/4(Thrust Desired) -> Saturation/1
  Saturation/1 -> Display/1, Thrust/1
  Saturation1/1 -> Pitch/1
  Saturation2/1 -> Roll/1
  LQR/3(Yaw rate Desired) -> Yawrate/1
  Meaured Yaw/1 -> Subsystem1/5(Measured Yaw), Subsystem/5(Measured Yaw), Gain1/1
  Subsystem/1(Xb Error) -> xbe int/1, LQR/1(xe)
  Subsystem/2(Yb Error) -> ybe int/1, LQR/2(ye)
  Demux/1 -> Subsystem/1(X)  "Traj X"
  Demux/2 -> Subsystem/3(Y)  "Traj Y"
  Demux1/1 -> Subsystem/2(Measured X)  "Mesured X"
  Demux1/2 -> Subsystem/4(Measured Y)  "Measured Y"
  [ze] -> LQR/3(ze)
  Gain1/1 -> Subtract1/2
  Gain/1 -> Subtract1/1
  Subtract1/1 -> [yawe]
  [yawe] -> LQR/7("yawe ")
  xbe int/1 -> LQR/8(xe int)
  ybe int/1 -> LQR/9(ye int)
  ze int/1 -> [ze_int]
  [ze_int] -> LQR/10(ze int)
  Subtract/1 -> ze int/1, [ze]
  "Trajdot "/1 -> Demux2/1
  Demux2/1 -> Subsystem1/1(Xdot)
  Demux2/2 -> Subsystem1/3(Ydot)
  Demux1/4 -> Subsystem1/2(Measured Xdot)
  Demux1/5 -> Subsystem1/4(Measured Ydot)
  Demux1/6 -> Subtract2/2
  Subsystem1/1(Xdotb Error) -> [xdote]
  Subsystem1/2(Ydotb Error) -> [ydote]
  [xdote] -> LQR/4(xdote)
  [ydote] -> LQR/5(ydote)
  Demux2/3 -> Subtract2/1
  Subtract2/1 -> [zdote]
  [zdote] -> LQR/6(zdote)

== system crazyflie/Off-board PID Position Controller ==
  Traj : Inport
  Position State : Inport  Port=2
  Meaured Yaw : Inport  Port=3
  Demux : Demux
  Demux1 : Demux  Outputs=6
  Display : Display
  Display1 : Display
  Gain : Gain
  Gain1 : Gain  Gain=180/pi
  Saturation : Saturate  UpperLimit=60000  LowerLimit=1000
  Saturation1 : Saturate  UpperLimit=30  LowerLimit=-30
  Saturation2 : Saturate  UpperLimit=30  LowerLimit=-30
  Subsystem : Subsystem
  Terminator : Terminator
  Terminator1 : Terminator
  Terminator2 : Terminator
  X PID : Subsystem
  Y PID : Subsystem
  Yaw PID : Subsystem
  Z PID : Subsystem
  Roll : Outport
  Pitch : Outport  Port=2
  Yawrate : Outport  Port=3
  Thrust : Outport  Port=4
  wires:
  Traj/1 -> Demux/1
  X PID/1(X PID) -> Saturation1/1
  Demux/4 -> Z PID/1(Z)  "Traj Z"
  Demux/3 -> Gain/1  "Traj Yaw"
  Position State/1 -> Demux1/1
  Demux1/4 -> Terminator/1
  Demux1/5 -> Terminator1/1
  Demux1/6 -> Terminator2/1
  Demux1/3 -> Z PID/2(Measured Z)  "Measured Z"
  Y PID/1(Y PID) -> Saturation2/1
  Z PID/1(Z PID) -> Saturation/1
  Saturation/1 -> Display/1, Thrust/1
  Saturation1/1 -> Pitch/1, Display1/1
  Saturation2/1 -> Roll/1
  Yaw PID/1(Yaw PID) -> Yawrate/1
  Meaured Yaw/1 -> Subsystem/5(Measured Yaw), Gain1/1
  Gain/1 -> Yaw PID/1(Yaw)
  Gain1/1 -> Yaw PID/2(Measured Yaw)
  Subsystem/1(Xb Error) -> X PID/1(Xb Error)
  Subsystem/2(Yb Error) -> Y PID/1(Yb Error)
  Demux/1 -> Subsystem/1(X)  "Traj X"
  Demux/2 -> Subsystem/3(Y)  "Traj Y"
  Demux1/1 -> Subsystem/2(Measured X)  "Mesured X"
  Demux1/2 -> Subsystem/4(Measured Y)  "Measured Y"

== system crazyflie/Off-board PID Position Controller1 ==
  Traj : Inport
  Position State : Inport  Port=2
  Meaured Yaw : Inport  Port=3
  Demux : Demux
  Demux1 : Demux  Outputs=3
  Display : Display
  Display1 : Display
  Gain : Gain
  Gain1 : Gain  Gain=180/pi
  Saturation : Saturate  UpperLimit=60000  LowerLimit=1000
  Saturation1 : Saturate  UpperLimit=30  LowerLimit=-30
  Saturation2 : Saturate  UpperLimit=30  LowerLimit=-30
  Subsystem : Subsystem
  X PID : Subsystem
  Y PID : Subsystem
  Yaw PID : Subsystem
  Z PID : Subsystem
  Roll : Outport
  Pitch : Outport  Port=2
  Yawrate : Outport  Port=3
  Thrust : Outport  Port=4
  wires:
  Traj/1 -> Demux/1
  X PID/1(X PID) -> Saturation1/1
  Demux/4 -> Z PID/1(Z)  "Traj Z"
  Demux/3 -> Gain/1  "Traj Yaw"
  Position State/1 -> Demux1/1
  Demux1/3 -> Z PID/2(Measured Z)  "Measured Z"
  Y PID/1(Y PID) -> Saturation2/1
  Z PID/1(Z PID) -> Saturation/1
  Saturation/1 -> Display/1, Thrust/1
  Saturation1/1 -> Pitch/1, Display1/1
  Saturation2/1 -> Roll/1
  Yaw PID/1(Yaw PID) -> Yawrate/1
  Meaured Yaw/1 -> Subsystem/5(Measured Yaw), Gain1/1
  Gain/1 -> Yaw PID/1(Yaw)
  Gain1/1 -> Yaw PID/2(Measured Yaw)
  Subsystem/1(Xb Error) -> X PID/1(Xb Error)
  Subsystem/2(Yb Error) -> Y PID/1(Yb Error)
  Demux/1 -> Subsystem/1(X)  "Traj X"
  Demux/2 -> Subsystem/3(Y)  "Traj Y"
  Demux1/1 -> Subsystem/2(Measured X)  "Mesured X"
  Demux1/2 -> Subsystem/4(Measured Y)  "Measured Y"

== system crazyflie/On-board Controller ==
  note: 500 Hz
  note: Map to desired
      | attitude rate
  note: 250 Hz
  Roll : Inport
  Pitch : Inport  Port=2
  Yawrate : Inport  Port=3
  Thrust : Inport  Port=4
  Attitude State : Inport  Port=5
  "Attitude Controller " : Subsystem
  Attitude Rate Controller : Subsystem
  Demux : Demux  Outputs=6
  Gain{,1,3..4} (4 alike) : Gain  Gain=180 / pi
  Gain2 : Gain  Gain=180/pi
  Gain5 : Gain  Gain=-1
  Mixer : Subsystem
  Terminator : Terminator
  "Yawrate Controller " : Subsystem
  Motor 1 : Outport
  Motor 2 : Outport  Port=2
  Motor 3 : Outport  Port=3
  Motor 4 : Outport  Port=4
  wires:
  Yawrate/1 -> "Yawrate Controller "/1(Desired Yawrate)
  Attitude Rate Controller/1(Commanded Roll) -> Mixer/1(Roll)
  Attitude Rate Controller/2(Commanded Pitch) -> Mixer/2(Pitch)
  "Yawrate Controller "/1(Commanded Yawrate) -> Gain5/1
  Thrust/1 -> Mixer/4(Thrust)
  Mixer/1(Motor 1) -> Motor 1/1
  Mixer/2(Motor 2) -> Motor 2/1
  Mixer/3(Motor 3) -> Motor 3/1
  Mixer/4(Motor 4) -> Motor 4/1
  Attitude State/1 -> Demux/1
  Demux/1 -> Gain1/1  "Measured Roll"
  Demux/2 -> Gain2/1  "Measured Pitch"
  Demux/4 -> Gain3/1  "Measured Roll Rate"
  Demux/5 -> Gain4/1  "Measured Pitch Rate"
  Demux/3 -> Terminator/1  "Yaw"
  Roll/1 -> "Attitude Controller "/1(Roll)
  Pitch/1 -> "Attitude Controller "/2(Pitch)
  "Attitude Controller "/1(Desired Roll) -> Attitude Rate Controller/1(Roll Rate)
  "Attitude Controller "/2("Desired Pitch ") -> Attitude Rate Controller/2(Pitch Rate)
  Gain/1 -> "Yawrate Controller "/2(Measured Yawrate)
  Demux/6 -> Gain/1  "Measured Yawrate"
  Gain1/1 -> "Attitude Controller "/3(Measured Roll)
  Gain2/1 -> "Attitude Controller "/4(Measured Pitch)
  Gain3/1 -> Attitude Rate Controller/3(Measured Roll Rate)
  Gain4/1 -> Attitude Rate Controller/4(Measured Pitch Rate)
  Gain5/1 -> Mixer/3(Yawrate)

== system crazyflie/On-board Controller1 ==
  note: 500 Hz
  note: Map to desired
      | attitude rate
  note: 250 Hz
  Roll : Inport
  Pitch : Inport  Port=2
  Yawrate : Inport  Port=3
  Thrust : Inport  Port=4
  Attitude State : Inport  Port=5
  "Attitude Controller " : Subsystem
  Attitude Rate Controller : Subsystem
  Demux : Demux  Outputs=6
  Gain{,1,3..4} (4 alike) : Gain  Gain=180 / pi
  Gain2 : Gain  Gain=180/pi
  Gain5 : Gain  Gain=-1
  Mixer : Subsystem
  Terminator : Terminator
  "Yawrate Controller " : Subsystem
  Motor 1 : Outport
  Motor 2 : Outport  Port=2
  Motor 3 : Outport  Port=3
  Motor 4 : Outport  Port=4
  wires:
  Yawrate/1 -> "Yawrate Controller "/1(Desired Yawrate)
  Attitude Rate Controller/1(Commanded Roll) -> Mixer/1(Roll)
  Attitude Rate Controller/2(Commanded Pitch) -> Mixer/2(Pitch)
  "Yawrate Controller "/1(Commanded Yawrate) -> Gain5/1
  Thrust/1 -> Mixer/4(Thrust)
  Mixer/1(Motor 1) -> Motor 1/1
  Mixer/2(Motor 2) -> Motor 2/1
  Mixer/3(Motor 3) -> Motor 3/1
  Mixer/4(Motor 4) -> Motor 4/1
  Attitude State/1 -> Demux/1
  Demux/1 -> Gain1/1  "Measured Roll"
  Demux/2 -> Gain2/1  "Measured Pitch"
  Demux/4 -> Gain3/1  "Measured Roll Rate"
  Demux/5 -> Gain4/1  "Measured Pitch Rate"
  Demux/3 -> Terminator/1  "Yaw"
  Roll/1 -> "Attitude Controller "/1(Roll)
  Pitch/1 -> "Attitude Controller "/2(Pitch)
  "Attitude Controller "/1(Desired Roll) -> Attitude Rate Controller/1(Roll Rate)
  "Attitude Controller "/2("Desired Pitch ") -> Attitude Rate Controller/2(Pitch Rate)
  Gain/1 -> "Yawrate Controller "/2(Measured Yawrate)
  Demux/6 -> Gain/1  "Measured Yawrate"
  Gain1/1 -> "Attitude Controller "/3(Measured Roll)
  Gain2/1 -> "Attitude Controller "/4(Measured Pitch)
  Gain3/1 -> Attitude Rate Controller/3(Measured Roll Rate)
  Gain4/1 -> Attitude Rate Controller/4(Measured Pitch Rate)
  Gain5/1 -> Mixer/3(Yawrate)

== system crazyflie/On-board Controller2 ==
  note: 500 Hz
  note: Map to desired
      | attitude rate
  note: 250 Hz
  Roll : Inport
  Pitch : Inport  Port=2
  Yawrate : Inport  Port=3
  Thrust : Inport  Port=4
  Attitude State : Inport  Port=5
  "Attitude Controller " : Subsystem
  Attitude Rate Controller : Subsystem
  Demux : Demux  Outputs=6
  Gain{,1,3..4} (4 alike) : Gain  Gain=180 / pi
  Gain2 : Gain  Gain=180/pi
  Gain5 : Gain  Gain=-1
  Mixer : Subsystem
  Terminator : Terminator
  "Yawrate Controller " : Subsystem
  Motor 1 : Outport
  Motor 2 : Outport  Port=2
  Motor 3 : Outport  Port=3
  Motor 4 : Outport  Port=4
  wires:
  Yawrate/1 -> "Yawrate Controller "/1(Desired Yawrate)
  Attitude Rate Controller/1(Commanded Roll) -> Mixer/1(Roll)
  Attitude Rate Controller/2(Commanded Pitch) -> Mixer/2(Pitch)
  "Yawrate Controller "/1(Commanded Yawrate) -> Gain5/1
  Thrust/1 -> Mixer/4(Thrust)
  Mixer/1(Motor 1) -> Motor 1/1
  Mixer/2(Motor 2) -> Motor 2/1
  Mixer/3(Motor 3) -> Motor 3/1
  Mixer/4(Motor 4) -> Motor 4/1
  Attitude State/1 -> Demux/1
  Demux/1 -> Gain1/1  "Measured Roll"
  Demux/2 -> Gain2/1  "Measured Pitch"
  Demux/4 -> Gain3/1  "Measured Roll Rate"
  Demux/5 -> Gain4/1  "Measured Pitch Rate"
  Demux/3 -> Terminator/1  "Yaw"
  Roll/1 -> "Attitude Controller "/1(Roll)
  Pitch/1 -> "Attitude Controller "/2(Pitch)
  "Attitude Controller "/1(Desired Roll) -> Attitude Rate Controller/1(Roll Rate)
  "Attitude Controller "/2("Desired Pitch ") -> Attitude Rate Controller/2(Pitch Rate)
  Gain/1 -> "Yawrate Controller "/2(Measured Yawrate)
  Demux/6 -> Gain/1  "Measured Yawrate"
  Gain1/1 -> "Attitude Controller "/3(Measured Roll)
  Gain2/1 -> "Attitude Controller "/4(Measured Pitch)
  Gain3/1 -> Attitude Rate Controller/3(Measured Roll Rate)
  Gain4/1 -> Attitude Rate Controller/4(Measured Pitch Rate)
  Gain5/1 -> Mixer/3(Yawrate)

== system crazyflie/On-board Controller3 ==
  note: 500 Hz
  note: Map to desired
      | attitude rate
  note: 250 Hz
  Roll : Inport
  Pitch : Inport  Port=2
  Yawrate : Inport  Port=3
  Thrust : Inport  Port=4
  Attitude State : Inport  Port=5
  "Attitude Controller " : Subsystem
  Attitude Rate Controller : Subsystem
  Demux : Demux  Outputs=6
  Gain{,1,3..4} (4 alike) : Gain  Gain=180 / pi
  Gain2 : Gain  Gain=180/pi
  Gain5 : Gain  Gain=-1
  Mixer : Subsystem
  Terminator : Terminator
  "Yawrate Controller " : Subsystem
  Motor 1 : Outport
  Motor 2 : Outport  Port=2
  Motor 3 : Outport  Port=3
  Motor 4 : Outport  Port=4
  wires:
  Yawrate/1 -> "Yawrate Controller "/1(Desired Yawrate)
  Attitude Rate Controller/1(Commanded Roll) -> Mixer/1(Roll)
  Attitude Rate Controller/2(Commanded Pitch) -> Mixer/2(Pitch)
  "Yawrate Controller "/1(Commanded Yawrate) -> Gain5/1
  Thrust/1 -> Mixer/4(Thrust)
  Mixer/1(Motor 1) -> Motor 1/1
  Mixer/2(Motor 2) -> Motor 2/1
  Mixer/3(Motor 3) -> Motor 3/1
  Mixer/4(Motor 4) -> Motor 4/1
  Attitude State/1 -> Demux/1
  Demux/1 -> Gain1/1  "Measured Roll"
  Demux/2 -> Gain2/1  "Measured Pitch"
  Demux/4 -> Gain3/1  "Measured Roll Rate"
  Demux/5 -> Gain4/1  "Measured Pitch Rate"
  Demux/3 -> Terminator/1  "Yaw"
  Roll/1 -> "Attitude Controller "/1(Roll)
  Pitch/1 -> "Attitude Controller "/2(Pitch)
  "Attitude Controller "/1(Desired Roll) -> Attitude Rate Controller/1(Roll Rate)
  "Attitude Controller "/2("Desired Pitch ") -> Attitude Rate Controller/2(Pitch Rate)
  Gain/1 -> "Yawrate Controller "/2(Measured Yawrate)
  Demux/6 -> Gain/1  "Measured Yawrate"
  Gain1/1 -> "Attitude Controller "/3(Measured Roll)
  Gain2/1 -> "Attitude Controller "/4(Measured Pitch)
  Gain3/1 -> Attitude Rate Controller/3(Measured Roll Rate)
  Gain4/1 -> Attitude Rate Controller/4(Measured Pitch Rate)
  Gain5/1 -> Mixer/3(Yawrate)

== system crazyflie/On-board Controller4 ==
  note: 500 Hz
  note: Map to desired
      | attitude rate
  note: 250 Hz
  Roll : Inport
  Pitch : Inport  Port=2
  Yawrate : Inport  Port=3
  Thrust : Inport  Port=4
  Attitude State : Inport  Port=5
  "Attitude Controller " : Subsystem
  Attitude Rate Controller : Subsystem
  Demux : Demux  Outputs=6
  Gain{,1,3..4} (4 alike) : Gain  Gain=180 / pi
  Gain2 : Gain  Gain=180/pi
  Gain5 : Gain  Gain=-1
  Mixer : Subsystem
  Terminator : Terminator
  "Yawrate Controller " : Subsystem
  Motor 1 : Outport
  Motor 2 : Outport  Port=2
  Motor 3 : Outport  Port=3
  Motor 4 : Outport  Port=4
  wires:
  Yawrate/1 -> "Yawrate Controller "/1(Desired Yawrate)
  Attitude Rate Controller/1(Commanded Roll) -> Mixer/1(Roll)
  Attitude Rate Controller/2(Commanded Pitch) -> Mixer/2(Pitch)
  "Yawrate Controller "/1(Commanded Yawrate) -> Gain5/1
  Thrust/1 -> Mixer/4(Thrust)
  Mixer/1(Motor 1) -> Motor 1/1
  Mixer/2(Motor 2) -> Motor 2/1
  Mixer/3(Motor 3) -> Motor 3/1
  Mixer/4(Motor 4) -> Motor 4/1
  Attitude State/1 -> Demux/1
  Demux/1 -> Gain1/1  "Measured Roll"
  Demux/2 -> Gain2/1  "Measured Pitch"
  Demux/4 -> Gain3/1  "Measured Roll Rate"
  Demux/5 -> Gain4/1  "Measured Pitch Rate"
  Demux/3 -> Terminator/1  "Yaw"
  Roll/1 -> "Attitude Controller "/1(Roll)
  Pitch/1 -> "Attitude Controller "/2(Pitch)
  "Attitude Controller "/1(Desired Roll) -> Attitude Rate Controller/1(Roll Rate)
  "Attitude Controller "/2("Desired Pitch ") -> Attitude Rate Controller/2(Pitch Rate)
  Gain/1 -> "Yawrate Controller "/2(Measured Yawrate)
  Demux/6 -> Gain/1  "Measured Yawrate"
  Gain1/1 -> "Attitude Controller "/3(Measured Roll)
  Gain2/1 -> "Attitude Controller "/4(Measured Pitch)
  Gain3/1 -> Attitude Rate Controller/3(Measured Roll Rate)
  Gain4/1 -> Attitude Rate Controller/4(Measured Pitch Rate)
  Gain5/1 -> Mixer/3(Yawrate)

== system crazyflie/PWM to RPM ==
  Motor 1 : Inport
  Motor 2 : Inport  Port=2
  Motor 3 : Inport  Port=3
  Motor 4 : Inport  Port=4
  Display{,1..3} (4 alike) : Display
  Polynomial{,1..3} (4 alike) : Polyval  Coefs=[1.6809E-19 -3.0288E-14 2.0739E-09 -6.7596E-05 1.3515E+00 0]
  RPM 1 : Outport
  RPM 2 : Outport  Port=2
  RPM 3 : Outport  Port=3
  RPM 4 : Outport  Port=4
  wires:
  Motor 1/1 -> Polynomial/1
  Polynomial/1 -> Display/1, RPM 1/1
  Motor 2/1 -> Polynomial1/1
  Polynomial1/1 -> Display1/1, RPM 2/1
  Motor 3/1 -> Polynomial2/1
  Polynomial2/1 -> Display2/1, RPM 3/1
  Motor 4/1 -> Polynomial3/1
  Polynomial3/1 -> Display3/1, RPM 4/1

== system crazyflie/PWM to RPM1 ==
  Motor 1 : Inport
  Motor 2 : Inport  Port=2
  Motor 3 : Inport  Port=3
  Motor 4 : Inport  Port=4
  Display{,1..3} (4 alike) : Display
  Polynomial{,1..3} (4 alike) : Polyval  Coefs=[1.6809E-19 -3.0288E-14 2.0739E-09 -6.7596E-05 1.3515E+00 0]
  RPM 1 : Outport
  RPM 2 : Outport  Port=2
  RPM 3 : Outport  Port=3
  RPM 4 : Outport  Port=4
  wires:
  Motor 1/1 -> Polynomial/1
  Polynomial/1 -> Display/1, RPM 1/1
  Motor 2/1 -> Polynomial1/1
  Polynomial1/1 -> Display1/1, RPM 2/1
  Motor 3/1 -> Polynomial2/1
  Polynomial2/1 -> Display2/1, RPM 3/1
  Motor 4/1 -> Polynomial3/1
  Polynomial3/1 -> Display3/1, RPM 4/1

== system crazyflie/PWM to RPM2 ==
  Motor 1 : Inport
  Motor 2 : Inport  Port=2
  Motor 3 : Inport  Port=3
  Motor 4 : Inport  Port=4
  Display{,1..3} (4 alike) : Display
  Polynomial{,1..3} (4 alike) : Polyval  Coefs=[1.6809E-19 -3.0288E-14 2.0739E-09 -6.7596E-05 1.3515E+00 0]
  RPM 1 : Outport
  RPM 2 : Outport  Port=2
  RPM 3 : Outport  Port=3
  RPM 4 : Outport  Port=4
  wires:
  Motor 1/1 -> Polynomial/1
  Polynomial/1 -> Display/1, RPM 1/1
  Motor 2/1 -> Polynomial1/1
  Polynomial1/1 -> Display1/1, RPM 2/1
  Motor 3/1 -> Polynomial2/1
  Polynomial2/1 -> Display2/1, RPM 3/1
  Motor 4/1 -> Polynomial3/1
  Polynomial3/1 -> Display3/1, RPM 4/1

== system crazyflie/PWM to RPM3 ==
  Motor 1 : Inport
  Motor 2 : Inport  Port=2
  Motor 3 : Inport  Port=3
  Motor 4 : Inport  Port=4
  Display{,1..3} (4 alike) : Display
  Polynomial{,1..3} (4 alike) : Polyval  Coefs=[1.6809E-19 -3.0288E-14 2.0739E-09 -6.7596E-05 1.3515E+00 0]
  RPM 1 : Outport
  RPM 2 : Outport  Port=2
  RPM 3 : Outport  Port=3
  RPM 4 : Outport  Port=4
  wires:
  Motor 1/1 -> Polynomial/1
  Polynomial/1 -> Display/1, RPM 1/1
  Motor 2/1 -> Polynomial1/1
  Polynomial1/1 -> Display1/1, RPM 2/1
  Motor 3/1 -> Polynomial2/1
  Polynomial2/1 -> Display2/1, RPM 3/1
  Motor 4/1 -> Polynomial3/1
  Polynomial3/1 -> Display3/1, RPM 4/1

== system crazyflie/PWM to RPM4 ==
  Motor 1 : Inport
  Motor 2 : Inport  Port=2
  Motor 3 : Inport  Port=3
  Motor 4 : Inport  Port=4
  Display{,1..3} (4 alike) : Display
  Polynomial{,1..3} (4 alike) : Polyval  Coefs=[1.6809E-19 -3.0288E-14 2.0739E-09 -6.7596E-05 1.3515E+00 0]
  RPM 1 : Outport
  RPM 2 : Outport  Port=2
  RPM 3 : Outport  Port=3
  RPM 4 : Outport  Port=4
  wires:
  Motor 1/1 -> Polynomial/1
  Polynomial/1 -> Display/1, RPM 1/1
  Motor 2/1 -> Polynomial1/1
  Polynomial1/1 -> Display1/1, RPM 2/1
  Motor 3/1 -> Polynomial2/1
  Polynomial2/1 -> Display2/1, RPM 3/1
  Motor 4/1 -> Polynomial3/1
  Polynomial3/1 -> Display3/1, RPM 4/1

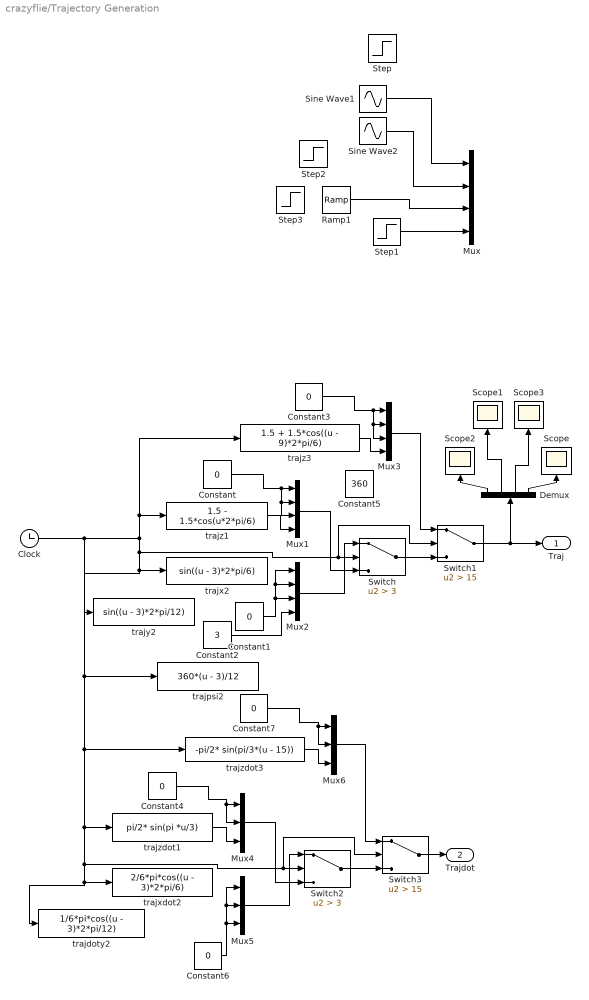
== system crazyflie/Trajectory Generation ==
  Clock : Clock
  Constant{,1,3..4,6..7} (6 alike) : Constant  Value=0
  Constant2 : Constant  Value=3
  Constant5 : Constant  Value=360
  Demux : Demux
  Mux{,1..3} (4 alike) : Mux
  Mux4 : Mux  Inputs=3
  Mux5 : Mux  Inputs=3
  Mux6 : Mux  Inputs=3
  Ramp1 : simulink/Sources/Ramp  slope=1  start=5  X0=0
  Scope{,1..3} (4 alike) : Scope
  Sine Wave1 : Sin  Frequency=pi/10  Phase=-pi/2  SampleTime=0
  Sine Wave2 : Sin  Frequency=pi/10  SampleTime=0
  Step : Step  Time=10  SampleTime=0
  Step1 : Step  SampleTime=0
  Step2 : Step  Time=5  SampleTime=0
  Step3 : Step  Time=15  After=60  SampleTime=0
  Switch : Switch  Criteria=u2 > Threshold  Threshold=3
  Switch1 : Switch  Criteria=u2 > Threshold  Threshold=15
  Switch2 : Switch  Criteria=u2 > Threshold  Threshold=3
  Switch3 : Switch  Criteria=u2 > Threshold  Threshold=15
  trajdoty2 : Fcn  Expr=1/6*pi*cos((u - 3)*2*pi/12)
  trajpsi2 : Fcn  Expr=360*(u - 3)/12
  "trajx2 " : Fcn  Expr=sin((u - 3)*2*pi/6)
  trajxdot2 : Fcn  Expr=2/6*pi*cos((u - 3)*2*pi/6)
  trajy2 : Fcn  Expr=sin((u - 3)*2*pi/12)
  "trajz1 " : Fcn  Expr=1.5 - 1.5*cos(u*2*pi/6)
  trajz3 : Fcn  Expr=1.5 + 1.5*cos((u - 9)*2*pi/6)
  "trajzdot1 " : Fcn  Expr=pi/2* sin(pi *u/3)
  trajzdot3 : Fcn  Expr=-pi/2* sin(pi/3*(u - 15))
  Traj : Outport
  Trajdot : Outport  Port=2
  wires:
  Step1/1 -> Mux/4
  Sine Wave1/1 -> Mux/1
  Sine Wave2/1 -> Mux/2
  Ramp1/1 -> Mux/3
  Constant/1 -> Mux1/3, Mux1/2, Mux1/1
  Mux1/1 -> Switch/3
  Mux2/1 -> Switch/1
  Switch/1 -> Switch1/3
  Constant3/1 -> Mux3/3, Mux3/2, Mux3/1
  Mux3/1 -> Switch1/1
  "trajzdot1 "/1 -> Mux4/3
  Constant4/1 -> Mux4/2, Mux4/1
  Clock/1 -> trajpsi2/1, Switch3/2, Switch2/2, trajdoty2/1, trajxdot2/1, "trajzdot1 "/1, trajzdot3/1, Switch1/2, Switch/2, trajy2/1, "trajx2 "/1, trajz3/1, "trajz1 "/1
  Mux4/1 -> Switch2/3
  Mux5/1 -> Switch2/1
  Constant6/1 -> Mux5/1, Mux5/2, Mux5/3
  Switch2/1 -> Switch3/3
  trajzdot3/1 -> Mux6/3
  Constant7/1 -> Mux6/2, Mux6/1
  Mux6/1 -> Switch3/1
  Switch3/1 -> Trajdot/1
  Switch1/1 -> Demux/1, Traj/1
  Demux/1 -> Scope2/1
  Demux/2 -> Scope1/1
  Demux/3 -> Scope3/1
  trajz3/1 -> Mux3/4
  "trajz1 "/1 -> Mux1/4
  Constant2/1 -> Mux2/4
  Demux/4 -> Scope/1
  Constant1/1 -> Mux2/3, Mux2/2, Mux2/1

== system crazyflie/Off-board ILQR Position Controller/ILQR ==
  x meas : Inport
  y meas : Inport  Port=2
  z meas : Inport  Port=3
  xdot meas : Inport  Port=4
  ydot meas : Inport  Port=5
  zdot meas : Inport  Port=6
  "yaw meas " : Inport  Port=7
  traj : Inport  Port=8
  trajdot : Inport  Port=9
  Constant1 : Constant  Value=9.81*0.041
  Demux : Demux
  Demux1 : Demux  Outputs=3
  Demux2 : Demux
  Fcn : Fcn  Expr=-86876*u^2+154046*u
  MATLAB Function : MATLAB Function  TreatAsAtomicUnit=on
  Memory : Memory  X0=[0 0 0 0]'
  Mux : Mux  Inputs=7
  Mux1 : Mux  Inputs=7
  Saturation : Saturate  UpperLimit=0.65  LowerLimit=0
  Scope : Scope
  Scope1 : Scope
  Sum : Sum  Inputs=|++
  Roll Desired : Outport
  Pitch Desired : Outport  Port=2
  Yaw rate Desired : Outport  Port=3
  Thrust Desired : Outport  Port=4
  wires:
  x meas/1 -> Mux/1
  y meas/1 -> Mux/2
  Fcn/1 -> Thrust Desired/1
  z meas/1 -> Mux/3
  ydot meas/1 -> Mux/5
  zdot meas/1 -> Mux/6
  "yaw meas "/1 -> Mux/7
  xdot meas/1 -> Mux/4
  Sum/1 -> Saturation/1
  Constant1/1 -> Sum/2
  traj/1 -> Demux/1
  trajdot/1 -> Demux1/1
  Mux/1 -> MATLAB Function/1(state)
  Mux1/1 -> MATLAB Function/2(setpoint)
  Demux/1 -> Mux1/1  "trjax"
  Demux/2 -> Mux1/2  "trajy"
  Demux/4 -> Mux1/3  "trajz"
  Demux1/1 -> Mux1/4  "trajxdot"
  Demux1/2 -> Mux1/5  "trajydot"
  Demux1/3 -> Mux1/6  "trajzdot"
  Demux/3 -> Mux1/7  "trajpsi"
  MATLAB Function/1(u_new) -> Demux2/1, Memory/1
  Memory/1 -> MATLAB Function/3(u_prev)
  Demux2/1 -> Roll Desired/1
  Demux2/2 -> Pitch Desired/1
  Demux2/4 -> Yaw rate Desired/1, Scope1/1
  Demux2/3 -> Sum/1
  Saturation/1 -> Scope/1, Fcn/1
